simulink model "SAGE-Simulink"  (R2022b)
settings: Solver=VariableStepAuto  StartTime=0.0  StopTime=2  RelTol=1e-3
libraries: spsSeriesRLCBranchLib x12, spsVoltageMeasurementLib x4, spsDCVoltageSourceLib x3, spsCurrentMeasurementLib x3, spsDiodeLib x1, spsGroundLib x1, spsIdealSwitchLib x1, spsMosfetLib x1, eePwmGenerator x1, spspowerguiLib x1
settings Model: Creator=gobis  LastModifiedBy=gobis

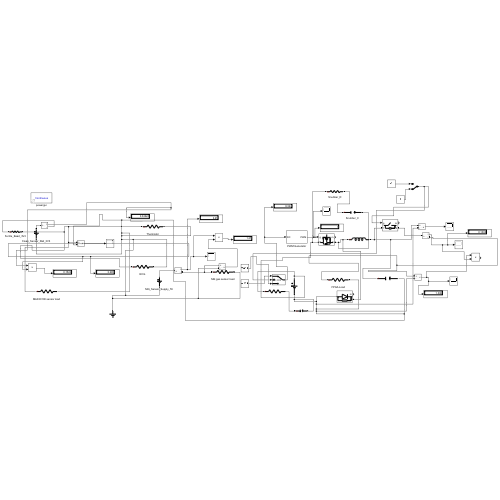
[thumbnail: Simulink's stored preview of the top-level diagram]
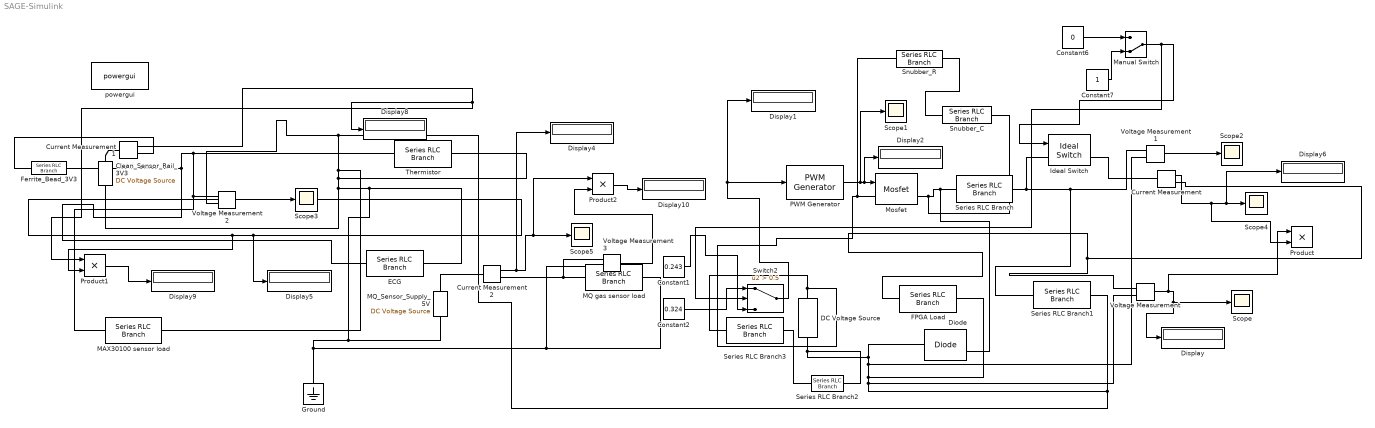
== system SAGE-Simulink ==
  Clean_Sensor_Rail_3V3 : spsDCVoltageSourceLib/DC Voltage Source  Amplitude=3.3  Measurements=None
  Constant1 : Constant  Value=0.243
  Constant2 : Constant  Value=0.324
  Constant6 : Constant  Value=0
  Constant7 : Constant
  Current Measurement : spsCurrentMeasurementLib/Current Measurement  PhasorSimulation=off  OutputType=Complex  PSBequivalent=0
  Current Measurement1 : spsCurrentMeasurementLib/Current Measurement  PhasorSimulation=off  OutputType=Complex  PSBequivalent=0
  Current Measurement2 : spsCurrentMeasurementLib/Current Measurement  PhasorSimulation=off  OutputType=Complex  PSBequivalent=0
  DC Voltage Source : spsDCVoltageSourceLib/DC Voltage Source  Amplitude=3.7  Measurements=None
  Diode : spsDiodeLib/Diode  Ron=0.001  Lon=0  Vf=0.8  IC=0  UseSnubber=0  Rs=500  Cs=250e-9  Measurements=on
  Display{,1..2,4..6,8..10} (9 alike) : Display
  ECG : spsSeriesRLCBranchLib/Series RLC Branch  LConnTagsString=__new0  RConnTagsString=__new0  BranchType=R  Resistance=330  Inductance=1e-3  SetiL0=off  InitialCurrent=0  Capacitance=1e-6  Setx0=off  InitialVoltage=0  Measurements=None
  FPGA Load : spsSeriesRLCBranchLib/Series RLC Branch  LConnTagsString=__new0  RConnTagsString=__new0  BranchType=R  Resistance=10  Inductance=1e-3  SetiL0=off  InitialCurrent=0  Capacitance=1e-6  Setx0=off  InitialVoltage=0  Measurements=None
  Ferrite_Bead_3V3 : spsSeriesRLCBranchLib/Series RLC Branch  LConnTagsString=__new0  RConnTagsString=__new0  BranchType=R  Resistance=0.1  Inductance=1e-3  SetiL0=off  InitialCurrent=0  Capacitance=1e-6  Setx0=off  InitialVoltage=0  Measurements=None
  Ground : spsGroundLib/Ground  LConnTagsString=a
  Ideal Switch : spsIdealSwitchLib/Ideal Switch  Ron=0.001  Lon=0  IC=0  Rs=1e5  Cs=inf  Measurements=on
  MAX30100 sensor load : spsSeriesRLCBranchLib/Series RLC Branch  LConnTagsString=__new0  RConnTagsString=__new0  BranchType=R  Resistance=100  Inductance=1e-3  SetiL0=off  InitialCurrent=0  Capacitance=1e-6  Setx0=off  InitialVoltage=0  Measurements=None
  MQ gas sensor load : spsSeriesRLCBranchLib/Series RLC Branch  LConnTagsString=__new0  RConnTagsString=__new0  BranchType=R  Resistance=20  Inductance=1e-3  SetiL0=off  InitialCurrent=0  Capacitance=1e-6  Setx0=off  InitialVoltage=0  Measurements=None
  MQ_Sensor_Supply_5V : spsDCVoltageSourceLib/DC Voltage Source  Amplitude=5  Measurements=None
  Manual Switch : ManualSwitch  CurrentSetting=0
  Mosfet : spsMosfetLib/Mosfet  Ron=0.1  Lon=0  Rd=0.01  Vfd=0  IC=0  Rs=1e5  Cs=inf  Measurements=on
  PWM Generator : eePwmGenerator/PWM Generator  CarrCount=Up  Tper=5e-5  Tdelay=0  Ts=0
  Product : Product
  Product1 : Product
  Product2 : Product
  Scope{,1..5} (6 alike) : Scope
  Series RLC Branch : spsSeriesRLCBranchLib/Series RLC Branch  LConnTagsString=__new0  RConnTagsString=__new0  BranchType=L  Resistance=1  Inductance=100e-6  SetiL0=off  InitialCurrent=0  Capacitance=1e-6  Setx0=off  InitialVoltage=0  Measurements=None
  Series RLC Branch1 : spsSeriesRLCBranchLib/Series RLC Branch  LConnTagsString=__new0  RConnTagsString=__new0  BranchType=C  Resistance=1  Inductance=1e-3  SetiL0=off  InitialCurrent=0  Capacitance=470e-6  Setx0=off  InitialVoltage=0  Measurements=None
  Series RLC Branch2 : spsSeriesRLCBranchLib/Series RLC Branch  LConnTagsString=__new0  RConnTagsString=__new0  BranchType=C  Resistance=1  Inductance=1e-3  SetiL0=off  InitialCurrent=0  Capacitance=100e-6  Setx0=off  InitialVoltage=0  Measurements=None
  Series RLC Branch3 : spsSeriesRLCBranchLib/Series RLC Branch  LConnTagsString=__new0  RConnTagsString=__new0  BranchType=R  Resistance=0.01  Inductance=1e-3  SetiL0=off  InitialCurrent=0  Capacitance=1e-6  Setx0=off  InitialVoltage=0  Measurements=None
  Snubber_C : spsSeriesRLCBranchLib/Series RLC Branch  LConnTagsString=__new0  RConnTagsString=__new0  BranchType=C  Resistance=1  Inductance=1e-3  SetiL0=off  InitialCurrent=0  Capacitance=10e-9  Setx0=off  InitialVoltage=0  Measurements=None
  Snubber_R : spsSeriesRLCBranchLib/Series RLC Branch  LConnTagsString=__new0  RConnTagsString=__new0  BranchType=R  Resistance=10  Inductance=1e-3  SetiL0=off  InitialCurrent=0  Capacitance=1e-6  Setx0=off  InitialVoltage=0  Measurements=None
  Switch2 : Switch  Criteria=u2 > Threshold  Threshold=0.5  SaturateOnIntegerOverflow=off  InputSameDT=off
  Thermistor : spsSeriesRLCBranchLib/Series RLC Branch  LConnTagsString=__new0  RConnTagsString=__new0  BranchType=R  Resistance=1000  Inductance=1e-3  SetiL0=off  InitialCurrent=0  Capacitance=1e-6  Setx0=off  InitialVoltage=0  Measurements=None
  Voltage Measurement{,1..3} (4 alike) : spsVoltageMeasurementLib/Voltage Measurement  PhasorSimulation=off  OutputType=Complex  PSBequivalent=0
  powergui : spspowerguiLib/powergui  Priority=1  SimulationMode=Continuous  SampleTime=50e-6  frequency=60  Iterations=50  frequencyindice=0  Pbase=100e6  ErrMax=1e-4  UnitsV=kV  UnitsW=MW  buscounter=0  FunctionMessages=off  echomessages=off  EnableUseOfTLC=off  CurrentSourceSwitches=off  DisableSnubberDevices=off  DisableRonSwitches=off  DisableVfSwitches=off  DisplayEquations=off  AutomaticDiscreteSolvers=off  SolverType=Tustin/Backward Euler (TBE)  Interpol=off  ExternalGateDelay=off  methode=off  Ts=100  x0status=blocks  SPID=on  SwTol=0  HookPort=off  NonlinearTolerance=1e-4  nMaxIteration=100  ContinueOnMaxIteration=off  RestoreLinks=warning  ResistiveCurrentMeasurement=off  Frange=[0:2:500]  Ylog=off  Xlog=on  ShowGrid=off  save=off  variable=ZData  structure=0  ZoomFFT=off  StartTime=0.0  cycles=1  DisplayStyle=1  fundamental=60  FreqAxis=off  MaxFrequency=1000  frequencyindicesteady=1  RmsSteady=1  display=off
  wires:
  Constant7/1 -> Manual Switch/2
  Constant6/1 -> Manual Switch/1
  Voltage Measurement1/1 -> Scope2/1
  Switch2/1 -> Display1/1, PWM Generator/1
  Current Measurement1/1 -> Display8/1, Product1/1
  PWM Generator/1 -> Scope1/1, Display2/1, Mosfet/1
  Manual Switch/1 -> Ideal Switch/1, Switch2/2
  Constant1/1 -> Switch2/3
  Constant2/1 -> Switch2/1
  Voltage Measurement/1 -> Product/1, Display/1, Scope/1
  Voltage Measurement2/1 -> Scope3/1, Product1/2, Display5/1
  Product1/1 -> Display9/1
  Current Measurement/1 -> Product/2, Display6/1, Scope4/1
  Current Measurement2/1 -> Display4/1, Product2/1, Scope5/1
  Voltage Measurement3/1 -> Product2/2
  Product2/1 -> Display10/1
  connections:
  Ferrite_Bead_3V3/RConn1 -- Thermistor/LConn1 -- MAX30100 sensor load/LConn1 -- Voltage Measurement2/LConn1 -- ECG/LConn1
  Voltage Measurement/LConn2 -- Series RLC Branch1/RConn1 -- Voltage Measurement2/LConn2 -- Clean_Sensor_Rail_3V3/LConn1 -- ECG/RConn1 -- MQ gas sensor load/RConn1 -- Voltage Measurement3/LConn2 -- Ground/LConn1 -- MQ_Sensor_Supply_5V/LConn1 -- Thermistor/RConn1 -- MAX30100 sensor load/RConn1 -- FPGA Load/RConn1 -- Series RLC Branch2/RConn1 -- DC Voltage Source/LConn1 -- Diode/LConn1 -- Voltage Measurement1/LConn2
  Voltage Measurement1/LConn1 -- Series RLC Branch1/LConn1 -- Ideal Switch/LConn1 -- Series RLC Branch/RConn1
  Voltage Measurement/LConn1 -- FPGA Load/LConn1 -- Current Measurement/RConn1
  Series RLC Branch/LConn1 -- Snubber_C/RConn1 -- Mosfet/RConn1 -- Diode/RConn1
  Current Measurement1/LConn1 -- Clean_Sensor_Rail_3V3/RConn1
  Current Measurement/LConn1 -- Ideal Switch/RConn1
  DC Voltage Source/RConn1 -- Series RLC Branch3/LConn1 -- Snubber_R/LConn1 -- Mosfet/LConn1
  MQ_Sensor_Supply_5V/RConn1 -- Current Measurement2/LConn1
  Current Measurement2/RConn1 -- Voltage Measurement3/LConn1 -- MQ gas sensor load/LConn1
  Ferrite_Bead_3V3/LConn1 -- Current Measurement1/RConn1
  Snubber_R/RConn1 -- Snubber_C/LConn1
  Series RLC Branch2/LConn1 -- Series RLC Branch3/RConn1
